simulink model "system_sim_test4"  (R2015a)
settings: Solver=ode45  StartTime=0.0  StopTime=1000  FixedStep=1  RelTol=1e-3
libraries: simulink x1
settings Model: Creator=marco  LastModifiedBy=mrclpt
settings SolverCC: ZeroCrossControl=EnableAll

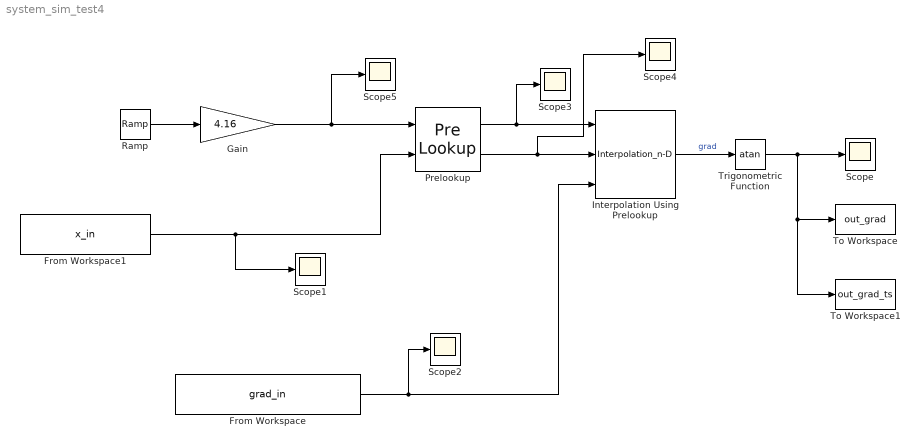
== system system_sim_test4 ==
  From Workspace : FromWorkspace  VariableName=grad_in  OutDataTypeStr=double  SampleTime=0  OutputAfterFinalValue=Setting to zero
  From Workspace1 : FromWorkspace  VariableName=x_in  OutDataTypeStr=double  SampleTime=0  OutputAfterFinalValue=Setting to zero
  Gain : Gain  Gain=4.16
  Interpolation Using Prelookup : Interpolation_n-D  NumberOfTableDimensions=1  TableSource=Input port  InternalRulePriority=Speed
      settings: InputPortMap=u0,u1,p2
  Prelookup : PreLookup  BreakpointsDataSource=Input port  BreakpointsData=[10:10:110]  ExtrapMethod=Linear
      settings: InputPortMap=u0,p1
  Ramp : simulink/Sources/Ramp  slope=1  start=0  X0=0
  Scope{,1..5} (6 alike) : Scope
      Scope2 settings: SaveName=ScopeData2
      Scope3 settings: SaveName=ScopeData3
      Scope4 settings: SaveName=ScopeData4
      Scope5 settings: SaveName=ScopeData5
  To Workspace : ToWorkspace  VariableName=out_grad  SampleTime=-1
      settings: Save2DSignal=2-D array (concatenate along first dimension)
  To Workspace1 : ToWorkspace  VariableName=out_grad_ts  SaveFormat=Timeseries  SampleTime=-1
      settings: Save2DSignal=2-D array (concatenate along first dimension)
  Trigonometric Function : Trigonometry  Operator=atan
  wires:
  Interpolation Using Prelookup/1 -> Trigonometric Function/1  "grad"
  Prelookup/1 -> Scope3/1, Interpolation Using Prelookup/1
  Prelookup/2 -> Scope4/1, Interpolation Using Prelookup/2
  From Workspace/1 -> Scope2/1, Interpolation Using Prelookup/3
  From Workspace1/1 -> Scope1/1, Prelookup/2
  Trigonometric Function/1 -> To Workspace1/1, To Workspace/1, Scope/1
  Ramp/1 -> Gain/1
  Gain/1 -> Scope5/1, Prelookup/1
